simulink model "SimscapeCrane_MPChard"  (R2015b)
settings: Solver=ode15s  StartTime=0.0  StopTime=T  RelTol=1e-3
values from neighbouring files (symbols this model uses):
  m = m1/N    [ConstraintMatrices.m]
  N = N1/(n+c)    [SoftPadding.m]    (also in testMPC.m = ceil(Tf/Ts); testMyLP.m = ceil(1.5/Ts); testRHC.m = ceil(1.5/Ts))
  s = size(A)    [Prediction.m]
  Ts = 1.5/10    (= 0.15)    [testMPC.m]    (also in testMyLP.m; testRHC.m)
  xTarget = [xRange(2)*0.8 0 xRange(2)*0.8 0 0 0 0 0]'    [testMyLP.m]
  xZero = xRange(2)*0.05    [testMPC.m]    (also in testRHC.m = 0)
  yZero = yRange(2)*0.05    [testMPC.m]    (also in testRHC.m = 0)
undefined symbols (not defined in the file or in its folder): Al, blx0, blxe, CD, Dx0, MR, TxBreak, TxCoulomb, TxVisc, TyBreak, TyCoulomb, TzBreak, TzCoulomb, ucon, X, xRange, Y, yRange, Z, zRange, zZero
undefined symbols (not defined in the file): M, TorqueMultX, TorqueMultY, TorqueMultZ, TxTrans, TyTrans, TyVisc, TzTrans, TzVisc
libraries: sm_lib x146, fl_lib x62, nesl_utility x24, elec_lib x9, simulink x6, sm_double_wishbone_suspension_lib x4, aerolibtransform2 x1
(part 13 of 14)

== system SimscapeCrane_MPChard/Crane1/XY actuator/DC Y ==
  DCYcontrolSignal : Inport
  " Lead Screw" : fl_lib/Mechanical/Mechanisms/Wheel and Axle  R=2 cm  or=1  orient=1  t_specify=off  t_priority=High  t=0 N*m  f_specify=off  f_priority=High  f=0 N
  DC Motor2 : elec_lib/Actuators & Drivers/Rotational Actuators/DC Motor  parameterization=2  Ra=3.9 Ohm  La=1.2e-5 H  emf_or_torque=1  Kv=7.2e-5 V/rpm  Ki=6.876e-4 N*m/A  T_stall=10000 mN*m  w_max=190 rpm  w_rated=190 rpm  P_rated=0.08 W  V_rated=24 V  J=0.01 g*cm^2  lam_param=1  lam=0 N*m/(rad/s)  i_noload=0 A  V_i_noload=1.5 V  speed0=0 rpm  alpha=0.00393 1/K  Tmeas=25 C  thermal_mass=100 J/K  initial_temperature=25 C
  Force Sensor : fl_lib/Mechanical/Mechanical Sensors/Ideal Force Sensor
  Gear Box : fl_lib/Mechanical/Mechanisms/Gear Box  Tag=Factory Generic  ratio=1/30  t_in_specify=off  t_in_priority=High  t_in=0 N*m  t_out_specify=off  t_out_priority=High  t_out=0 N*m
  Mechanical Rotational Reference1 : fl_lib/Mechanical/Rotational Elements/Mechanical Rotational Reference
  Mechanical Translational Reference4 : fl_lib/Mechanical/Translational Elements/Mechanical Translational Reference
  PS Gain : fl_lib/Physical Signals/Functions/PS Gain  gain=-1*Uy
  PWM & H-Bridge1 : Subsystem
  SL2V_1 : Subsystem
  Conn1 : PMIOPort  Port=1  Side=Right
  wires:
  DCYcontrolSignal/1 -> SL2V_1/1(SL)
  connections:
  Force Sensor/RConn2 -- PS Gain/LConn1
  Mechanical Translational Reference4/LConn1 -- Force Sensor/LConn1
  Mechanical Rotational Reference1/LConn1 -- DC Motor2/RConn2
  Gear Box/RConn1 -- " Lead Screw"/LConn1
  Force Sensor/RConn1 -- " Lead Screw"/RConn1
  DC Motor2/LConn2 -- Gear Box/LConn1
  PWM & H-Bridge1/RConn2 -- DC Motor2/RConn1
  SL2V_1/RConn2 -- PWM & H-Bridge1/LConn2
  SL2V_1/RConn3 -- PWM & H-Bridge1/LConn3
  SL2V_1/RConn4 -- PWM & H-Bridge1/LConn4
  SL2V_1/RConn1 -- PWM & H-Bridge1/LConn1
  PWM & H-Bridge1/RConn1 -- DC Motor2/LConn1
  Conn1/RConn1 -- PS Gain/RConn1

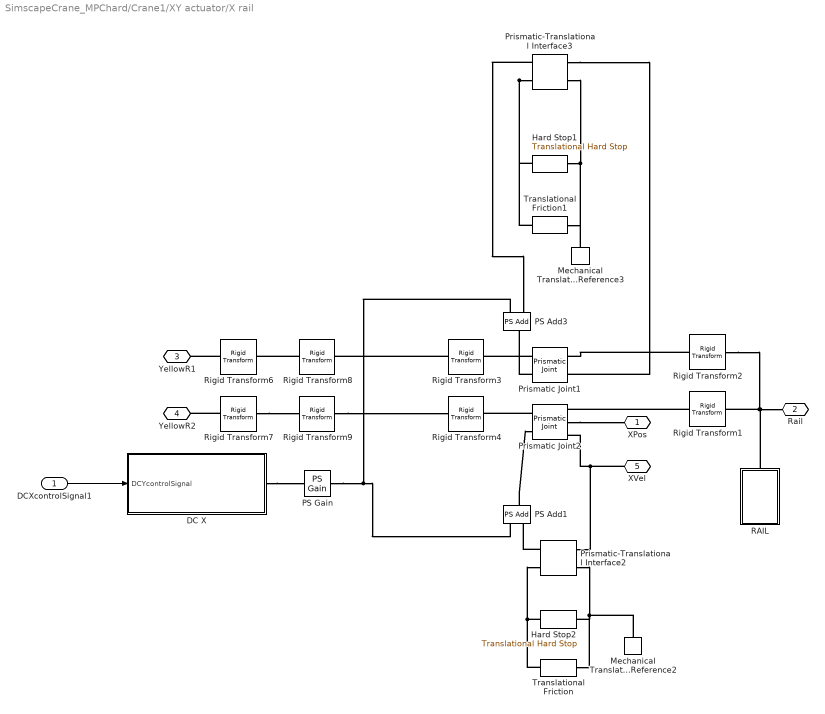
== system SimscapeCrane_MPChard/Crane1/XY actuator/X rail ==
  DCXcontrolSignal1 : Inport
  DC X : Subsystem
  Hard Stop1 : fl_lib/Mechanical/Translational Elements/Translational Hard Stop  upper_bnd=-xZero +xRange(2) m  lower_bnd=(xRange(1)-xZero) m  stiff_up=2e6 N/m  stiff_low=2e6 N/m  D_up=1000 N/(m/s)  D_low=1000 N/(m/s)  v_specify=off  v_priority=High  v=0 m/s  f_specify=off  f_priority=High  f=0 N  x_specify=off  x_priority=High  x=1 cm
  Hard Stop2 : fl_lib/Mechanical/Translational Elements/Translational Hard Stop  upper_bnd=-xZero +xRange(2) m  lower_bnd=(xRange(1)-xZero) m  stiff_up=2e6 N/m  stiff_low=2e6 N/m  D_up=1000 N/(m/s)  D_low=1000 N/(m/s)  v_specify=off  v_priority=High  v=0 m/s  f_specify=off  f_priority=High  f=0 N  x_specify=off  x_priority=High  x=1 cm
  Mechanical Translational Reference2 : fl_lib/Mechanical/Translational Elements/Mechanical Translational Reference
  Mechanical Translational Reference3 : fl_lib/Mechanical/Translational Elements/Mechanical Translational Reference
  PS Add1 : fl_lib/Physical Signals/Functions/PS Add
  PS Add3 : fl_lib/Physical Signals/Functions/PS Add
  PS Gain : fl_lib/Physical Signals/Functions/PS Gain  gain=1/2
  Prismatic Joint1 : sm_lib/Joints/Prismatic Joint  SenseConstraintForce=off  SenseConstraintForceX=off  SenseConstraintForceY=off  SenseConstraintForceZ=off  SenseConstraintTorque=off  SenseConstraintTorqueX=off  SenseConstraintTorqueY=off  SenseConstraintTorqueZ=off  SenseTotalForce=off  SenseTotalForceX=off  SenseTotalForceY=off  SenseTotalForceZ=off  SenseTotalTorque=off  SenseTotalTorqueX=off  SenseTotalTorqueY=off  SenseTotalTorqueZ=off  CompositeWrenchDir=FollowerOnBase  CompositeWrenchFrame=BaseFrame  EquilibriumPosition=0  EquilibriumPositionUnits=m  SpringStiffness=0  SpringStiffnessUnits=N/m  DampingCoefficient=0  DampingCoefficientUnits=N/(m/s)  TorqueActuationMode=InputTorque  MotionActuationMode=ComputedMotion  SensePosition=off  SenseVelocity=on  SenseAcceleration=off  SenseTorqueForce=off  PositionTargetSpecify=off  PositionTargetPriority=High  PositionTargetValue=0  PositionTargetValueUnits=m  VelocityTargetSpecify=off  VelocityTargetPriority=High  VelocityTargetValue=0  VelocityTargetValueUnits=m/s  BlockFunction=simmechanics.library.joints.prismatic_joint
  Prismatic Joint2 : sm_lib/Joints/Prismatic Joint  SenseConstraintForce=off  SenseConstraintForceX=off  SenseConstraintForceY=off  SenseConstraintForceZ=off  SenseConstraintTorque=off  SenseConstraintTorqueX=off  SenseConstraintTorqueY=off  SenseConstraintTorqueZ=off  SenseTotalForce=off  SenseTotalForceX=off  SenseTotalForceY=off  SenseTotalForceZ=off  SenseTotalTorque=off  SenseTotalTorqueX=off  SenseTotalTorqueY=off  SenseTotalTorqueZ=off  CompositeWrenchDir=FollowerOnBase  CompositeWrenchFrame=BaseFrame  EquilibriumPosition=0  EquilibriumPositionUnits=m  SpringStiffness=0  SpringStiffnessUnits=N/m  DampingCoefficient=0  DampingCoefficientUnits=N/(m/s)  TorqueActuationMode=InputTorque  MotionActuationMode=ComputedMotion  SensePosition=on  SenseVelocity=on  SenseAcceleration=off  SenseTorqueForce=off  PositionTargetSpecify=off  PositionTargetPriority=High  PositionTargetValue=0  PositionTargetValueUnits=m  VelocityTargetSpecify=off  VelocityTargetPriority=High  VelocityTargetValue=0  VelocityTargetValueUnits=m/s  BlockFunction=simmechanics.library.joints.prismatic_joint
  Prismatic-Translational Interface2 : sm_double_wishbone_suspension_lib/Testing Platform/Prismatic-Translational Interface
  Prismatic-Translational Interface3 : sm_double_wishbone_suspension_lib/Testing Platform/Prismatic-Translational Interface
  "RAIL " : Subsystem
  Rigid Transform1 : sm_lib/Frames and Transforms/Rigid Transform  TranslationMethod=Cartesian  TranslationLengthUnit=m  TranslationStandardAxis=+Z  TranslationStandardOffset=0  TranslationCartesianOffset="[0 0.5  0]"  TranslationROffset=0  TranslationROffsetUnits=m  TranslationZOffset=0  TranslationZOffsetUnits=m  TranslationThetaOffset=0  TranslationThetaOffsetUnits=deg  RotationMethod=StandardAxis  RotationAngleUnits=deg  RotationStandardAxis=-Y  RotationAngle=90  RotationArbitraryAxis=[0 0 1]  FollAlignAxisA=+X  BaseAlignAxisA=+Y  FollAlignAxisB=+Y  BaseAlignAxisB=+Z  RotationSequenceAxes=FollowerAxes  RotationSequence=XYX  RotationSequenceAngles=[0 0 0]  RotationSequenceAnglesUnits=deg  RotationMatrix=[1 0 0; 0 1 0; 0 0 1]  BlockFunction=simmechanics.library.frames_transforms.rigid_transform
  Rigid Transform2 : sm_lib/Frames and Transforms/Rigid Transform  TranslationMethod=Cartesian  TranslationLengthUnit=m  TranslationStandardAxis=+Z  TranslationStandardOffset=0  TranslationCartesianOffset="[ 0 -0.5  0]"  TranslationROffset=0  TranslationROffsetUnits=m  TranslationZOffset=0  TranslationZOffsetUnits=m  TranslationThetaOffset=0  TranslationThetaOffsetUnits=deg  RotationMethod=StandardAxis  RotationAngleUnits=deg  RotationStandardAxis=-Y  RotationAngle=90  RotationArbitraryAxis=[0 0 1]  FollAlignAxisA=+X  BaseAlignAxisA=+Y  FollAlignAxisB=+Y  BaseAlignAxisB=+Z  RotationSequenceAxes=FollowerAxes  RotationSequence=XYX  RotationSequenceAngles=[0 0 0]  RotationSequenceAnglesUnits=deg  RotationMatrix=[1 0 0; 0 1 0; 0 0 1]  BlockFunction=simmechanics.library.frames_transforms.rigid_transform
  Rigid Transform3 : sm_lib/Frames and Transforms/Rigid Transform  TranslationMethod=None  TranslationLengthUnit=m  TranslationStandardAxis=+Z  TranslationStandardOffset=0  TranslationCartesianOffset="[0.5 1  0]"  TranslationROffset=0  TranslationROffsetUnits=m  TranslationZOffset=0  TranslationZOffsetUnits=m  TranslationThetaOffset=0  TranslationThetaOffsetUnits=deg  RotationMethod=StandardAxis  RotationAngleUnits=deg  RotationStandardAxis=+Y  RotationAngle=90  RotationArbitraryAxis=[0 0 1]  FollAlignAxisA=+X  BaseAlignAxisA=+Y  FollAlignAxisB=+Y  BaseAlignAxisB=+Z  RotationSequenceAxes=FollowerAxes  RotationSequence=XYX  RotationSequenceAngles=[0 0 0]  RotationSequenceAnglesUnits=deg  RotationMatrix=[1 0 0; 0 1 0; 0 0 1]  BlockFunction=simmechanics.library.frames_transforms.rigid_transform
  Rigid Transform4 : sm_lib/Frames and Transforms/Rigid Transform  TranslationMethod=None  TranslationLengthUnit=m  TranslationStandardAxis=+Z  TranslationStandardOffset=0  TranslationCartesianOffset="[0.5 1  0]"  TranslationROffset=0  TranslationROffsetUnits=m  TranslationZOffset=0  TranslationZOffsetUnits=m  TranslationThetaOffset=0  TranslationThetaOffsetUnits=deg  RotationMethod=StandardAxis  RotationAngleUnits=deg  RotationStandardAxis=+Y  RotationAngle=90  RotationArbitraryAxis=[0 0 1]  FollAlignAxisA=+X  BaseAlignAxisA=+Y  FollAlignAxisB=+Y  BaseAlignAxisB=+Z  RotationSequenceAxes=FollowerAxes  RotationSequence=XYX  RotationSequenceAngles=[0 0 0]  RotationSequenceAnglesUnits=deg  RotationMatrix=[1 0 0; 0 1 0; 0 0 1]  BlockFunction=simmechanics.library.frames_transforms.rigid_transform
  Rigid Transform6 : sm_lib/Frames and Transforms/Rigid Transform  TranslationMethod=Cartesian  TranslationLengthUnit=m  TranslationStandardAxis=+Z  TranslationStandardOffset=0  TranslationCartesianOffset="[-0.28 0  0]"  TranslationROffset=0  TranslationROffsetUnits=m  TranslationZOffset=0  TranslationZOffsetUnits=m  TranslationThetaOffset=0  TranslationThetaOffsetUnits=deg  RotationMethod=None  RotationAngleUnits=deg  RotationStandardAxis=+Y  RotationAngle=90  RotationArbitraryAxis=[0 0 1]  FollAlignAxisA=+X  BaseAlignAxisA=+Y  FollAlignAxisB=+Y  BaseAlignAxisB=+Z  RotationSequenceAxes=FollowerAxes  RotationSequence=XYX  RotationSequenceAngles=[0 0 0]  RotationSequenceAnglesUnits=deg  RotationMatrix=[1 0 0; 0 1 0; 0 0 1]  BlockFunction=simmechanics.library.frames_transforms.rigid_transform
  Rigid Transform7 : sm_lib/Frames and Transforms/Rigid Transform  TranslationMethod=Cartesian  TranslationLengthUnit=m  TranslationStandardAxis=+Z  TranslationStandardOffset=0  TranslationCartesianOffset="[-0.28 0  0]"  TranslationROffset=0  TranslationROffsetUnits=m  TranslationZOffset=0  TranslationZOffsetUnits=m  TranslationThetaOffset=0  TranslationThetaOffsetUnits=deg  RotationMethod=None  RotationAngleUnits=deg  RotationStandardAxis=+Y  RotationAngle=90  RotationArbitraryAxis=[0 0 1]  FollAlignAxisA=+X  BaseAlignAxisA=+Y  FollAlignAxisB=+Y  BaseAlignAxisB=+Z  RotationSequenceAxes=FollowerAxes  RotationSequence=XYX  RotationSequenceAngles=[0 0 0]  RotationSequenceAnglesUnits=deg  RotationMatrix=[1 0 0; 0 1 0; 0 0 1]  BlockFunction=simmechanics.library.frames_transforms.rigid_transform
  Rigid Transform8 : sm_lib/Frames and Transforms/Rigid Transform  TranslationMethod=Cartesian  TranslationLengthUnit=m  TranslationStandardAxis=+Z  TranslationStandardOffset=0  TranslationCartesianOffset="[xZero 0  0]"  TranslationROffset=0  TranslationROffsetUnits=m  TranslationZOffset=0  TranslationZOffsetUnits=m  TranslationThetaOffset=0  TranslationThetaOffsetUnits=deg  RotationMethod=None  RotationAngleUnits=deg  RotationStandardAxis=+Y  RotationAngle=90  RotationArbitraryAxis=[0 0 1]  FollAlignAxisA=+X  BaseAlignAxisA=+Y  FollAlignAxisB=+Y  BaseAlignAxisB=+Z  RotationSequenceAxes=FollowerAxes  RotationSequence=XYX  RotationSequenceAngles=[0 0 0]  RotationSequenceAnglesUnits=deg  RotationMatrix=[1 0 0; 0 1 0; 0 0 1]  BlockFunction=simmechanics.library.frames_transforms.rigid_transform
  Rigid Transform9 : sm_lib/Frames and Transforms/Rigid Transform  TranslationMethod=Cartesian  TranslationLengthUnit=m  TranslationStandardAxis=+Z  TranslationStandardOffset=0  TranslationCartesianOffset="[xZero 0  0]"  TranslationROffset=0  TranslationROffsetUnits=m  TranslationZOffset=0  TranslationZOffsetUnits=m  TranslationThetaOffset=0  TranslationThetaOffsetUnits=deg  RotationMethod=None  RotationAngleUnits=deg  RotationStandardAxis=+Y  RotationAngle=90  RotationArbitraryAxis=[0 0 1]  FollAlignAxisA=+X  BaseAlignAxisA=+Y  FollAlignAxisB=+Y  BaseAlignAxisB=+Z  RotationSequenceAxes=FollowerAxes  RotationSequence=XYX  RotationSequenceAngles=[0 0 0]  RotationSequenceAnglesUnits=deg  RotationMatrix=[1 0 0; 0 1 0; 0 0 1]  BlockFunction=simmechanics.library.frames_transforms.rigid_transform
  Translational Friction : fl_lib/Mechanical/Translational Elements/Translational Friction  brkwy_frc=(TxBreak+TxCoulomb)/2 N  Col_frc=TxCoulomb/2 N  visc_coef=TxVisc/2 N/(m/s)  trans_coef=TxTrans s/m  vel_thr=1e-4 m/s  v_specify=off  v_priority=None  v=0 m/s  f_specify=off  f_priority=None  f=0 N
  Translational Friction1 : fl_lib/Mechanical/Translational Elements/Translational Friction  brkwy_frc=(TxBreak+TxCoulomb)/2 N  Col_frc=TxCoulomb/2 N  visc_coef=TxVisc/2 N/(m/s)  trans_coef=TxTrans s/m  vel_thr=1e-4 m/s  v_specify=off  v_priority=None  v=0 m/s  f_specify=off  f_priority=None  f=0 N
  XPos : PMIOPort  Port=1  Side=Right
  Rail : PMIOPort  Port=2  Side=Right
  YellowR1 : PMIOPort  Port=3  Side=Left
  YellowR2 : PMIOPort  Port=4  Side=Left
  XVel : PMIOPort  Port=5  Side=Right
  wires:
  DCXcontrolSignal1/1 -> DC X/1(DCYcontrolSignal)
  connections:
  Rigid Transform7/RConn1 -- Rigid Transform9/LConn1
  Rigid Transform6/LConn1 -- YellowR1/RConn1
  Prismatic Joint2/RConn2 -- XPos/RConn1
  Rigid Transform2/LConn1 -- Prismatic Joint1/RConn1
  Rigid Transform1/LConn1 -- Prismatic Joint2/RConn1
  "RAIL "/RConn1 -- Rigid Transform1/RConn1 -- Rigid Transform2/RConn1 -- Rail/RConn1
  Prismatic-Translational Interface2/LConn1 -- Prismatic Joint2/RConn3 -- XVel/RConn1
  Prismatic Joint1/LConn1 -- Rigid Transform3/RConn1
  Prismatic Joint2/LConn1 -- Rigid Transform4/RConn1
  PS Gain/RConn1 -- PS Add3/LConn2 -- PS Add1/LConn1
  DC X/RConn1 -- PS Gain/LConn1
  PS Add1/RConn1 -- Prismatic Joint2/LConn2
  Prismatic-Translational Interface2/RConn1 -- PS Add1/LConn2
  Prismatic Joint1/LConn2 -- PS Add3/RConn1
  Prismatic-Translational Interface3/LConn2 -- Hard Stop1/LConn1 -- Translational Friction1/LConn1 -- Mechanical Translational Reference3/LConn1
  Prismatic-Translational Interface3/RConn2 -- Hard Stop1/RConn1 -- Translational Friction1/RConn1
  Prismatic-Translational Interface3/RConn1 -- PS Add3/LConn1
  Prismatic-Translational Interface3/LConn1 -- Prismatic Joint1/RConn2
  Mechanical Translational Reference2/LConn1 -- Prismatic-Translational Interface2/LConn2 -- Hard Stop2/LConn1 -- Translational Friction/LConn1
  Hard Stop2/RConn1 -- Translational Friction/RConn1 -- Prismatic-Translational Interface2/RConn2
  Rigid Transform3/LConn1 -- Rigid Transform8/RConn1
  Rigid Transform7/LConn1 -- YellowR2/RConn1
  Rigid Transform8/LConn1 -- Rigid Transform6/RConn1
  Rigid Transform9/RConn1 -- Rigid Transform4/LConn1

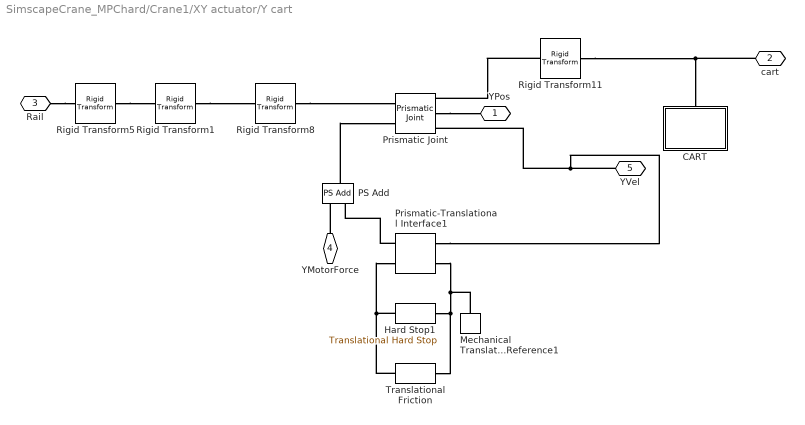
== system SimscapeCrane_MPChard/Crane1/XY actuator/Y cart ==
  CART : Subsystem
  Hard Stop1 : fl_lib/Mechanical/Translational Elements/Translational Hard Stop  upper_bnd=-yZero +yRange(2) m  lower_bnd=(yRange(1)-yZero) m  stiff_up=2e6 N/m  stiff_low=2e6 N/m  D_up=1000 N/(m/s)  D_low=1000 N/(m/s)  v_specify=off  v_priority=High  v=0 m/s  f_specify=off  f_priority=High  f=0 N  x_specify=off  x_priority=High  x=1 cm
  Mechanical Translational Reference1 : fl_lib/Mechanical/Translational Elements/Mechanical Translational Reference
  PS Add : fl_lib/Physical Signals/Functions/PS Add
  Prismatic Joint : sm_lib/Joints/Prismatic Joint  SenseConstraintForce=off  SenseConstraintForceX=off  SenseConstraintForceY=off  SenseConstraintForceZ=off  SenseConstraintTorque=off  SenseConstraintTorqueX=off  SenseConstraintTorqueY=off  SenseConstraintTorqueZ=off  SenseTotalForce=off  SenseTotalForceX=off  SenseTotalForceY=off  SenseTotalForceZ=off  SenseTotalTorque=off  SenseTotalTorqueX=off  SenseTotalTorqueY=off  SenseTotalTorqueZ=off  CompositeWrenchDir=BaseOnFollower  CompositeWrenchFrame=BaseFrame  EquilibriumPosition=0  EquilibriumPositionUnits=m  SpringStiffness=0  SpringStiffnessUnits=N/m  DampingCoefficient=0  DampingCoefficientUnits=N/(m/s)  TorqueActuationMode=InputTorque  MotionActuationMode=ComputedMotion  SensePosition=on  SenseVelocity=on  SenseAcceleration=off  SenseTorqueForce=off  PositionTargetSpecify=on  PositionTargetPriority=High  PositionTargetValue=0  PositionTargetValueUnits=m  VelocityTargetSpecify=off  VelocityTargetPriority=High  VelocityTargetValue=0  VelocityTargetValueUnits=m/s  BlockFunction=simmechanics.library.joints.prismatic_joint
  Prismatic-Translational Interface1 : sm_double_wishbone_suspension_lib/Testing Platform/Prismatic-Translational Interface
  Rigid Transform1 : sm_lib/Frames and Transforms/Rigid Transform  TranslationMethod=Cartesian  TranslationLengthUnit=m  TranslationStandardAxis=+Z  TranslationStandardOffset=0  TranslationCartesianOffset="[0 yZero  0]"  TranslationROffset=0  TranslationROffsetUnits=m  TranslationZOffset=0  TranslationZOffsetUnits=m  TranslationThetaOffset=0  TranslationThetaOffsetUnits=deg  RotationMethod=None  RotationAngleUnits=deg  RotationStandardAxis=+Y  RotationAngle=90  RotationArbitraryAxis=[0 0 1]  FollAlignAxisA=+X  BaseAlignAxisA=+Y  FollAlignAxisB=+Y  BaseAlignAxisB=+Z  RotationSequenceAxes=FollowerAxes  RotationSequence=XYX  RotationSequenceAngles=[0 0 0]  RotationSequenceAnglesUnits=deg  RotationMatrix=[1 0 0; 0 1 0; 0 0 1]  BlockFunction=simmechanics.library.frames_transforms.rigid_transform
  Rigid Transform11 : sm_lib/Frames and Transforms/Rigid Transform  TranslationMethod=None  TranslationLengthUnit=m  TranslationStandardAxis=+Z  TranslationStandardOffset=0  TranslationCartesianOffset="[-0.5 0  0]"  TranslationROffset=0  TranslationROffsetUnits=m  TranslationZOffset=0  TranslationZOffsetUnits=m  TranslationThetaOffset=0  TranslationThetaOffsetUnits=deg  RotationMethod=StandardAxis  RotationAngleUnits=deg  RotationStandardAxis=+X  RotationAngle=90  RotationArbitraryAxis=[0 0 1]  FollAlignAxisA=+X  BaseAlignAxisA=+Y  FollAlignAxisB=+Y  BaseAlignAxisB=+Z  RotationSequenceAxes=FollowerAxes  RotationSequence=XYX  RotationSequenceAngles=[0 0 0]  RotationSequenceAnglesUnits=deg  RotationMatrix=[1 0 0; 0 1 0; 0 0 1]  BlockFunction=simmechanics.library.frames_transforms.rigid_transform
  Rigid Transform5 : sm_lib/Frames and Transforms/Rigid Transform  TranslationMethod=Cartesian  TranslationLengthUnit=m  TranslationStandardAxis=+Z  TranslationStandardOffset=0  TranslationCartesianOffset="[0 -0.3  0]"  TranslationROffset=0  TranslationROffsetUnits=m  TranslationZOffset=0  TranslationZOffsetUnits=m  TranslationThetaOffset=0  TranslationThetaOffsetUnits=deg  RotationMethod=None  RotationAngleUnits=deg  RotationStandardAxis=+Y  RotationAngle=90  RotationArbitraryAxis=[0 0 1]  FollAlignAxisA=+X  BaseAlignAxisA=+Y  FollAlignAxisB=+Y  BaseAlignAxisB=+Z  RotationSequenceAxes=FollowerAxes  RotationSequence=XYX  RotationSequenceAngles=[0 0 0]  RotationSequenceAnglesUnits=deg  RotationMatrix=[1 0 0; 0 1 0; 0 0 1]  BlockFunction=simmechanics.library.frames_transforms.rigid_transform
  Rigid Transform8 : sm_lib/Frames and Transforms/Rigid Transform  TranslationMethod=None  TranslationLengthUnit=m  TranslationStandardAxis=+Z  TranslationStandardOffset=0  TranslationCartesianOffset="[-0.5 0  0]"  TranslationROffset=0  TranslationROffsetUnits=m  TranslationZOffset=0  TranslationZOffsetUnits=m  TranslationThetaOffset=0  TranslationThetaOffsetUnits=deg  RotationMethod=StandardAxis  RotationAngleUnits=deg  RotationStandardAxis=-X  RotationAngle=90  RotationArbitraryAxis=[0 0 1]  FollAlignAxisA=+X  BaseAlignAxisA=+Y  FollAlignAxisB=+Y  BaseAlignAxisB=+Z  RotationSequenceAxes=FollowerAxes  RotationSequence=XYX  RotationSequenceAngles=[0 0 0]  RotationSequenceAnglesUnits=deg  RotationMatrix=[1 0 0; 0 1 0; 0 0 1]  BlockFunction=simmechanics.library.frames_transforms.rigid_transform
  Translational Friction : fl_lib/Mechanical/Translational Elements/Translational Friction  brkwy_frc=TyBreak+TyCoulomb N  Col_frc=TyCoulomb N  visc_coef=TyVisc N/(m/s)  trans_coef=TyTrans s/m  vel_thr=1e-4 m/s  v_specify=off  v_priority=None  v=0 m/s  f_specify=off  f_priority=None  f=0 N
  YPos : PMIOPort  Port=1  Side=Right
  cart : PMIOPort  Port=2  Side=Right
  Rail : PMIOPort  Port=3  Side=Left
  YMotorForce : PMIOPort  Port=4  Side=Left
  YVel : PMIOPort  Port=5  Side=Right
  connections:
  Rail/RConn1 -- Rigid Transform5/LConn1
  Prismatic Joint/RConn2 -- YPos/RConn1
  Rigid Transform11/RConn1 -- cart/RConn1 -- CART/RConn1
  Rigid Transform8/RConn1 -- Prismatic Joint/LConn1
  Rigid Transform11/LConn1 -- Prismatic Joint/RConn1
  YVel/RConn1 -- Prismatic-Translational Interface1/LConn1 -- Prismatic Joint/RConn3
  YMotorForce/RConn1 -- PS Add/LConn1
  PS Add/RConn1 -- Prismatic Joint/LConn2
  Translational Friction/RConn1 -- Hard Stop1/RConn1 -- Prismatic-Translational Interface1/RConn2
  Prismatic-Translational Interface1/LConn2 -- Hard Stop1/LConn1 -- Translational Friction/LConn1 -- Mechanical Translational Reference1/LConn1
  Prismatic-Translational Interface1/RConn1 -- PS Add/LConn2
  Rigid Transform1/RConn1 -- Rigid Transform8/LConn1
  Rigid Transform5/RConn1 -- Rigid Transform1/LConn1

== system SimscapeCrane_MPChard/Crane1/Frame/XMotorAesthetics/Motor ==
  Cart2 : sm_lib/Body Elements/Solid  InertiaType=PointMass  Mass=0  MassUnits=kg  CenterOfMass=[0 0 0]  CenterOfMassUnits=m  MomentsOfInertia=[1 1 1]  MomentsOfInertiaUnits=kg*m^2  ProductsOfInertia=[0 0 0]  ProductsOfInertiaUnits=kg*m^2  DensityBased=off  Density=1000  DensityUnits=kg/(m^3)  DoExposeReferenceFrame=on  SerializedFrames=<Frames/>  GraphicType=FromGeometry  MarkerShape=Sphere  MarkerSize=10  MarkerSizeUnits=m  GraphicVisPropType=AdvancedVisualProperties  GraphicDiffuseColor=[0.1 0.1 0.0]  GraphicSpecularColor=[0.5 0.5 0.5 1.0]  GraphicAmbientColor=[0.15 0.2 0.3 1.0]  GraphicEmissiveColor=[0.0 0.0 0.0 1.0]  GraphicShininess=30  GraphicOpacity=1.0  GeometryShape=Cylinder  RectangleSize=[1 1]  RectangleSizeUnits=m  BrickDimensions=[0.06 0.12 0.12]  BrickDimensionUnits=m  CylinderRadius=1.7  CylinderRadiusUnits=cm  CylinderLength=6  CylinderLengthUnits=cm  SphereRadius=1  SphereRadiusUnits=m  EllipsoidRadii=[1 1 1]  EllipsoidRadiiUnits=m  ExtrusionCrossSection=[1 1; -1 1; -1 -1; 1 -1]  ExtrusionCrossSectionUnits=m  ExtrusionLength=1  ExtrusionLengthUnits=m  PolygonNumSides=3  PolygonOuterRadius=1  PolygonOuterRadiusUnits=m  ExtGeomFileType=STL  ExtGeomFileUnits=m  RevolutionCrossSection=[1 1; 1 -1; 2 -1; 2 1]  RevolutionCrossSectionUnits=m  RevolutionExtent=Full  RevolutionAngle=180  RevolutionAngleUnits=deg  BlockFunction=simmechanics.library.body_elements.solid
  Cart3 : sm_lib/Body Elements/Solid  InertiaType=PointMass  Mass=0  MassUnits=kg  CenterOfMass=[0 0 0]  CenterOfMassUnits=m  MomentsOfInertia=[1 1 1]  MomentsOfInertiaUnits=kg*m^2  ProductsOfInertia=[0 0 0]  ProductsOfInertiaUnits=kg*m^2  DensityBased=off  Density=1000  DensityUnits=kg/(m^3)  DoExposeReferenceFrame=on  SerializedFrames=<Frames/>  GraphicType=FromGeometry  MarkerShape=Sphere  MarkerSize=10  MarkerSizeUnits=m  GraphicVisPropType=SimpleVisualProperties  GraphicDiffuseColor=[0.4 0.4 0.4]  GraphicSpecularColor=[0.5 0.5 0.5 1.0]  GraphicAmbientColor=[0.15 0.15 0.15 1.0]  GraphicEmissiveColor=[0.0 0.0 0.0 1.0]  GraphicShininess=75  GraphicOpacity=1.0  GeometryShape=Cylinder  RectangleSize=[1 1]  RectangleSizeUnits=m  BrickDimensions=[0.06 0.12 0.12]  BrickDimensionUnits=m  CylinderRadius=2.6  CylinderRadiusUnits=cm  CylinderLength=3  CylinderLengthUnits=cm  SphereRadius=1  SphereRadiusUnits=m  EllipsoidRadii=[1 1 1]  EllipsoidRadiiUnits=m  ExtrusionCrossSection=[1 1; -1 1; -1 -1; 1 -1]  ExtrusionCrossSectionUnits=m  ExtrusionLength=1  ExtrusionLengthUnits=m  PolygonNumSides=3  PolygonOuterRadius=1  PolygonOuterRadiusUnits=m  ExtGeomFileType=STL  ExtGeomFileUnits=m  RevolutionCrossSection=[1 1; 1 -1; 2 -1; 2 1]  RevolutionCrossSectionUnits=m  RevolutionExtent=Full  RevolutionAngle=180  RevolutionAngleUnits=deg  BlockFunction=simmechanics.library.body_elements.solid
  Rigid Transform3 : sm_lib/Frames and Transforms/Rigid Transform  TranslationMethod=None  TranslationLengthUnit=m  TranslationStandardAxis=-X  TranslationStandardOffset=0.04  TranslationCartesianOffset="[-0.5 0  0]"  TranslationROffset=0  TranslationROffsetUnits=m  TranslationZOffset=0  TranslationZOffsetUnits=m  TranslationThetaOffset=0  TranslationThetaOffsetUnits=deg  RotationMethod=StandardAxis  RotationAngleUnits=deg  RotationStandardAxis=-X  RotationAngle=90  RotationArbitraryAxis=[0 0 1]  FollAlignAxisA=+X  BaseAlignAxisA=+Y  FollAlignAxisB=+Y  BaseAlignAxisB=+Z  RotationSequenceAxes=FollowerAxes  RotationSequence=XYX  RotationSequenceAngles=[0 0 0]  RotationSequenceAnglesUnits=deg  RotationMatrix=[1 0 0; 0 1 0; 0 0 1]  BlockFunction=simmechanics.library.frames_transforms.rigid_transform
  Rigid Transform4 : sm_lib/Frames and Transforms/Rigid Transform  TranslationMethod=None  TranslationLengthUnit=m  TranslationStandardAxis=-X  TranslationStandardOffset=0.04  TranslationCartesianOffset="[-0.5 0  0]"  TranslationROffset=0  TranslationROffsetUnits=m  TranslationZOffset=0  TranslationZOffsetUnits=m  TranslationThetaOffset=0  TranslationThetaOffsetUnits=deg  RotationMethod=StandardAxis  RotationAngleUnits=deg  RotationStandardAxis=-X  RotationAngle=90  RotationArbitraryAxis=[0 0 1]  FollAlignAxisA=+X  BaseAlignAxisA=+Y  FollAlignAxisB=+Y  BaseAlignAxisB=+Z  RotationSequenceAxes=FollowerAxes  RotationSequence=XYX  RotationSequenceAngles=[0 0 0]  RotationSequenceAnglesUnits=deg  RotationMatrix=[1 0 0; 0 1 0; 0 0 1]  BlockFunction=simmechanics.library.frames_transforms.rigid_transform
  Rigid Transform5 : sm_lib/Frames and Transforms/Rigid Transform  TranslationMethod=StandardAxis  TranslationLengthUnit=m  TranslationStandardAxis=-Y  TranslationStandardOffset=0.015  TranslationCartesianOffset="[-0.5 0  0]"  TranslationROffset=0  TranslationROffsetUnits=m  TranslationZOffset=0  TranslationZOffsetUnits=m  TranslationThetaOffset=0  TranslationThetaOffsetUnits=deg  RotationMethod=None  RotationAngleUnits=deg  RotationStandardAxis=-X  RotationAngle=90  RotationArbitraryAxis=[0 0 1]  FollAlignAxisA=+X  BaseAlignAxisA=+Y  FollAlignAxisB=+Y  BaseAlignAxisB=+Z  RotationSequenceAxes=FollowerAxes  RotationSequence=XYX  RotationSequenceAngles=[0 0 0]  RotationSequenceAnglesUnits=deg  RotationMatrix=[1 0 0; 0 1 0; 0 0 1]  BlockFunction=simmechanics.library.frames_transforms.rigid_transform
  Rigid Transform6 : sm_lib/Frames and Transforms/Rigid Transform  TranslationMethod=StandardAxis  TranslationLengthUnit=m  TranslationStandardAxis=+Y  TranslationStandardOffset=0.03  TranslationCartesianOffset="[-0.5 0  0]"  TranslationROffset=0  TranslationROffsetUnits=m  TranslationZOffset=0  TranslationZOffsetUnits=m  TranslationThetaOffset=0  TranslationThetaOffsetUnits=deg  RotationMethod=None  RotationAngleUnits=deg  RotationStandardAxis=-X  RotationAngle=90  RotationArbitraryAxis=[0 0 1]  FollAlignAxisA=+X  BaseAlignAxisA=+Y  FollAlignAxisB=+Y  BaseAlignAxisB=+Z  RotationSequenceAxes=FollowerAxes  RotationSequence=XYX  RotationSequenceAngles=[0 0 0]  RotationSequenceAnglesUnits=deg  RotationMatrix=[1 0 0; 0 1 0; 0 0 1]  BlockFunction=simmechanics.library.frames_transforms.rigid_transform
  Conn1 : PMIOPort  Port=1  Side=Left
  connections:
  Rigid Transform3/RConn1 -- Cart2/RConn1
  Rigid Transform4/RConn1 -- Cart3/RConn1
  Rigid Transform5/LConn1 -- Rigid Transform6/LConn1 -- Conn1/RConn1
  Rigid Transform6/RConn1 -- Rigid Transform4/LConn1
  Rigid Transform5/RConn1 -- Rigid Transform3/LConn1

== system SimscapeCrane_MPChard/Crane1/XY actuator/DC Y/PWM & H-Bridge1 ==
  note: For validation purposes the simulation mode
      | can be set to PWM in both the Controlled PWM
      | and H-Bridge blocks.
  Controlled PWM Voltage : elec_lib/Actuators & Drivers/Drivers/Controlled PWM Voltage  F=10000 Hz  TD=0 s  pulse_width_offset=0 s  Vmin=0 V  Vmax=5 V  Vm=5 V  pwm_or_av=2  event_type=1  sample_time=1e-6 s
  Electrical Reference2 : fl_lib/Electrical/Electrical Elements/Electrical Reference
  H-Bridge : elec_lib/Actuators & Drivers/Drivers/H-Bridge  Venable=2.5 V  Vmax=5 V  Vreverse=2.5 V  Vbrake=2.5 V  Vm=24 V  pwm_or_av=2  discontinuous=0  freewheeling_mode=1  freewheeling_mode_disc=1  Ron=0.1 Ohm  Don=0.1 Ohm  Rload=10 Ohm  Lload=1e-5 H  F=10 kHz  thermal_mass=100 J/K  initial_temperature=298.15 K  Ron2=0.1 Ohm  Don2=0.05 Ohm  Tmeas=298.15 K  Tmeas2=398.15 K
  PWM Scope : Subsystem  Commented=on
  REV Scope : Subsystem  Commented=on
  Vr Scope : Subsystem  Commented=on
  V+ : PMIOPort  Port=1  Side=Right
  V- : PMIOPort  Port=2  Side=Right
  Vr : PMIOPort  Port=3  Side=Left
  REV : PMIOPort  Port=4  Side=Left
  "brk " : PMIOPort  Port=5  Side=Left
  "gnd " : PMIOPort  Port=6  Side=Left
  connections:
  V+/RConn1 -- H-Bridge/RConn1
  H-Bridge/RConn2 -- V-/RConn1 -- Electrical Reference2/LConn1
  PWM Scope/LConn1 -- H-Bridge/LConn1 -- Controlled PWM Voltage/RConn1
  Vr Scope/LConn1 -- Controlled PWM Voltage/LConn1 -- Vr/RConn1
  REV Scope/LConn1 -- H-Bridge/LConn3 -- REV/RConn1
  "gnd "/RConn1 -- H-Bridge/LConn2 -- Controlled PWM Voltage/RConn2 -- Controlled PWM Voltage/LConn2
  "brk "/RConn1 -- H-Bridge/LConn4

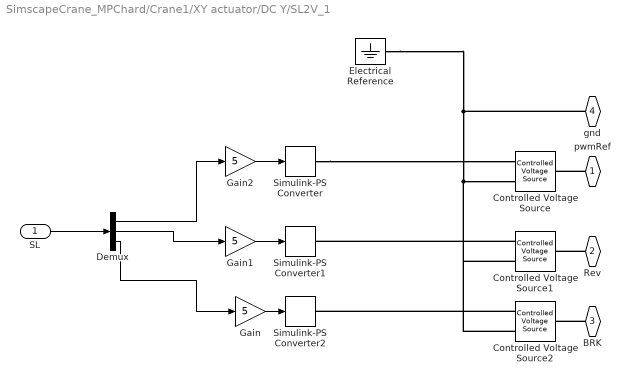
== system SimscapeCrane_MPChard/Crane1/XY actuator/DC Y/SL2V_1 ==
  SL : Inport
  Controlled Voltage Source : fl_lib/Electrical/Electrical Sources/Controlled Voltage Source
  Controlled Voltage Source1 : fl_lib/Electrical/Electrical Sources/Controlled Voltage Source
  Controlled Voltage Source2 : fl_lib/Electrical/Electrical Sources/Controlled Voltage Source
  Demux : Demux  Outputs=3
  Electrical Reference : fl_lib/Electrical/Electrical Elements/Electrical Reference
  Gain : Gain  Gain=5
  Gain1 : Gain  Gain=5
  Gain2 : Gain  Gain=5
  Simulink-PS Converter : nesl_utility/Simulink-PS Converter  PhysicalDomain=network_engine_domain  SubClassName=ps_input  LeftPortType=input  RightPortType=output  PseudoPeriodic=off  Frequencies=[]  NoiseDistribution=none  NoiseParameters=[]  Unit=V  AffineConversion=off  InputFiltering=off  SimscapeFilterOrder=1  InputFilterTimeConstant=.001  UdotUserProvided=0
  Simulink-PS Converter1 : nesl_utility/Simulink-PS Converter  PhysicalDomain=network_engine_domain  SubClassName=ps_input  LeftPortType=input  RightPortType=output  PseudoPeriodic=off  Frequencies=[]  NoiseDistribution=none  NoiseParameters=[]  Unit=V  AffineConversion=off  InputFiltering=off  SimscapeFilterOrder=1  InputFilterTimeConstant=.001  UdotUserProvided=0
  Simulink-PS Converter2 : nesl_utility/Simulink-PS Converter  PhysicalDomain=network_engine_domain  SubClassName=ps_input  LeftPortType=input  RightPortType=output  PseudoPeriodic=off  Frequencies=[]  NoiseDistribution=none  NoiseParameters=[]  Unit=V  AffineConversion=off  InputFiltering=off  SimscapeFilterOrder=1  InputFilterTimeConstant=.001  UdotUserProvided=0
  pwmRef : PMIOPort  Port=1  Side=Right
  Rev : PMIOPort  Port=2  Side=Right
  BRK : PMIOPort  Port=3  Side=Right
  "gnd " : PMIOPort  Port=4  Side=Right
  wires:
  SL/1 -> Demux/1
  Demux/1 -> Gain2/1
  Demux/3 -> Gain/1
  Gain/1 -> Simulink-PS Converter2/1
  Demux/2 -> Gain1/1
  Gain1/1 -> Simulink-PS Converter1/1
  Gain2/1 -> Simulink-PS Converter/1
  connections:
  Simulink-PS Converter/RConn1 -- Controlled Voltage Source/RConn1
  pwmRef/RConn1 -- Controlled Voltage Source/LConn1
  Electrical Reference/LConn1 -- Controlled Voltage Source/RConn2 -- Controlled Voltage Source1/RConn2 -- Controlled Voltage Source2/RConn2 -- "gnd "/RConn1
  Rev/RConn1 -- Controlled Voltage Source1/LConn1
  Controlled Voltage Source2/RConn1 -- Simulink-PS Converter2/RConn1
  BRK/RConn1 -- Controlled Voltage Source2/LConn1
  Controlled Voltage Source1/RConn1 -- Simulink-PS Converter1/RConn1

== system SimscapeCrane_MPChard/Crane1/XY actuator/X rail/DC X ==
  DCYcontrolSignal : Inport
  " Lead Screw" : fl_lib/Mechanical/Mechanisms/Wheel and Axle  R=2 cm  or=1  orient=1  t_specify=off  t_priority=High  t=0 N*m  f_specify=off  f_priority=High  f=0 N
  DC Motor2 : elec_lib/Actuators & Drivers/Rotational Actuators/DC Motor  parameterization=2  Ra=3.9 Ohm  La=1.2e-5 H  emf_or_torque=1  Kv=7.2e-5 V/rpm  Ki=6.876e-4 N*m/A  T_stall=10000 mN*m  w_max=190 rpm  w_rated=190 rpm  P_rated=0.08 W  V_rated=24 V  J=0.01 g*cm^2  lam_param=1  lam=0 N*m/(rad/s)  i_noload=0 A  V_i_noload=1.5 V  speed0=0 rpm  alpha=0.00393 1/K  Tmeas=25 C  thermal_mass=100 J/K  initial_temperature=25 C
  Force Sensor : fl_lib/Mechanical/Mechanical Sensors/Ideal Force Sensor
  Gear Box : fl_lib/Mechanical/Mechanisms/Gear Box  Tag=Factory Generic  ratio=1/30  t_in_specify=off  t_in_priority=High  t_in=0 N*m  t_out_specify=off  t_out_priority=High  t_out=0 N*m
  Mechanical Rotational Reference1 : fl_lib/Mechanical/Rotational Elements/Mechanical Rotational Reference
  Mechanical Translational Reference4 : fl_lib/Mechanical/Translational Elements/Mechanical Translational Reference
  PS Gain : fl_lib/Physical Signals/Functions/PS Gain  gain=-1*Ux
  PWM & H-Bridge : Subsystem
  SL2V_2 : Subsystem
  Conn1 : PMIOPort  Port=1  Side=Right
  wires:
  DCYcontrolSignal/1 -> SL2V_2/1(SL)
  connections:
  PS Gain/RConn1 -- Conn1/RConn1
  Mechanical Translational Reference4/LConn1 -- Force Sensor/LConn1
  Mechanical Rotational Reference1/LConn1 -- DC Motor2/RConn2
  Gear Box/RConn1 -- " Lead Screw"/LConn1
  Force Sensor/RConn1 -- " Lead Screw"/RConn1
  DC Motor2/LConn2 -- Gear Box/LConn1
  PWM & H-Bridge/RConn1 -- DC Motor2/LConn1
  PWM & H-Bridge/RConn2 -- DC Motor2/RConn1
  SL2V_2/RConn2 -- PWM & H-Bridge/LConn2
  SL2V_2/RConn3 -- PWM & H-Bridge/LConn3
  SL2V_2/RConn1 -- PWM & H-Bridge/LConn1
  SL2V_2/RConn4 -- PWM & H-Bridge/LConn4
  Force Sensor/RConn2 -- PS Gain/LConn1

== system SimscapeCrane_MPChard/Crane1/XY actuator/X rail/RAIL  ==
  Aesthetics : Subsystem
  Rail : sm_lib/Body Elements/Solid  InertiaType=CalculateFromGeometry  Mass=MR/2  MassUnits=kg  CenterOfMass=[0 0 0]  CenterOfMassUnits=m  MomentsOfInertia=[1 1 1]  MomentsOfInertiaUnits=kg*m^2  ProductsOfInertia=[0 0 0]  ProductsOfInertiaUnits=kg*m^2  DensityBased=off  Density=1000  DensityUnits=kg/(m^3)  DoExposeReferenceFrame=on  SerializedFrames=<Frames/>  GraphicType=FromGeometry  MarkerShape=Sphere  MarkerSize=10  MarkerSizeUnits=m  GraphicVisPropType=AdvancedVisualProperties  GraphicDiffuseColor=[0.0 0.0 0.0]  GraphicSpecularColor=[0.5 0.5 0.5 1.0]  GraphicAmbientColor=[0.15 0.15 0.15 1.0]  GraphicEmissiveColor=[0.0 0.0 0.0 1.0]  GraphicShininess=100  GraphicOpacity=1.0  GeometryShape=Brick  RectangleSize=[1 1]  RectangleSizeUnits=m  BrickDimensions=[1.2 0.04 0.04]  BrickDimensionUnits=m  CylinderRadius=0.02  CylinderRadiusUnits=m  CylinderLength=1  CylinderLengthUnits=m  SphereRadius=1  SphereRadiusUnits=m  EllipsoidRadii=[1 1 1]  EllipsoidRadiiUnits=m  ExtrusionCrossSection=[1 1; -1 1; -1 -1; 1 -1]  ExtrusionCrossSectionUnits=m  ExtrusionLength=1  ExtrusionLengthUnits=m  PolygonNumSides=3  PolygonOuterRadius=1  PolygonOuterRadiusUnits=m  ExtGeomFileType=STL  ExtGeomFileUnits=m  RevolutionCrossSection=[1 1; 1 -1; 2 -1; 2 1]  RevolutionCrossSectionUnits=m  RevolutionExtent=Full  RevolutionAngle=180  RevolutionAngleUnits=deg  BlockFunction=simmechanics.library.body_elements.solid
  Rail1 : sm_lib/Body Elements/Solid  InertiaType=CalculateFromGeometry  Mass=MR/2  MassUnits=kg  CenterOfMass=[0 0 0]  CenterOfMassUnits=m  MomentsOfInertia=[1 1 1]  MomentsOfInertiaUnits=kg*m^2  ProductsOfInertia=[0 0 0]  ProductsOfInertiaUnits=kg*m^2  DensityBased=off  Density=1000  DensityUnits=kg/(m^3)  DoExposeReferenceFrame=on  SerializedFrames=<Frames/>  GraphicType=FromGeometry  MarkerShape=Sphere  MarkerSize=10  MarkerSizeUnits=m  GraphicVisPropType=AdvancedVisualProperties  GraphicDiffuseColor=[0.0 0.0 0.0]  GraphicSpecularColor=[0.5 0.5 0.5 1.0]  GraphicAmbientColor=[0.15 0.15 0.15 1.0]  GraphicEmissiveColor=[0.0 0.0 0.0 1.0]  GraphicShininess=100  GraphicOpacity=1.0  GeometryShape=Brick  RectangleSize=[1 1]  RectangleSizeUnits=m  BrickDimensions=[1.2 0.04 0.04]  BrickDimensionUnits=m  CylinderRadius=0.02  CylinderRadiusUnits=m  CylinderLength=1  CylinderLengthUnits=m  SphereRadius=1  SphereRadiusUnits=m  EllipsoidRadii=[1 1 1]  EllipsoidRadiiUnits=m  ExtrusionCrossSection=[1 1; -1 1; -1 -1; 1 -1]  ExtrusionCrossSectionUnits=m  ExtrusionLength=1  ExtrusionLengthUnits=m  PolygonNumSides=3  PolygonOuterRadius=1  PolygonOuterRadiusUnits=m  ExtGeomFileType=STL  ExtGeomFileUnits=m  RevolutionCrossSection=[1 1; 1 -1; 2 -1; 2 1]  RevolutionCrossSectionUnits=m  RevolutionExtent=Full  RevolutionAngle=180  RevolutionAngleUnits=deg  BlockFunction=simmechanics.library.body_elements.solid
  Rigid Transform1 : sm_lib/Frames and Transforms/Rigid Transform  TranslationMethod=StandardAxis  TranslationLengthUnit=m  TranslationStandardAxis=-X  TranslationStandardOffset=0.04  TranslationCartesianOffset="[-0.5 0  0]"  TranslationROffset=0  TranslationROffsetUnits=m  TranslationZOffset=0  TranslationZOffsetUnits=m  TranslationThetaOffset=0  TranslationThetaOffsetUnits=deg  RotationMethod=None  RotationAngleUnits=deg  RotationStandardAxis=+Y  RotationAngle=90  RotationArbitraryAxis=[0 0 1]  FollAlignAxisA=+X  BaseAlignAxisA=+Y  FollAlignAxisB=+Y  BaseAlignAxisB=+Z  RotationSequenceAxes=FollowerAxes  RotationSequence=XYX  RotationSequenceAngles=[0 0 0]  RotationSequenceAnglesUnits=deg  RotationMatrix=[1 0 0; 0 1 0; 0 0 1]  BlockFunction=simmechanics.library.frames_transforms.rigid_transform
  Rigid Transform2 : sm_lib/Frames and Transforms/Rigid Transform  TranslationMethod=StandardAxis  TranslationLengthUnit=m  TranslationStandardAxis=+X  TranslationStandardOffset=0.04  TranslationCartesianOffset="[-0.5 0  0]"  TranslationROffset=0  TranslationROffsetUnits=m  TranslationZOffset=0  TranslationZOffsetUnits=m  TranslationThetaOffset=0  TranslationThetaOffsetUnits=deg  RotationMethod=None  RotationAngleUnits=deg  RotationStandardAxis=+Y  RotationAngle=90  RotationArbitraryAxis=[0 0 1]  FollAlignAxisA=+X  BaseAlignAxisA=+Y  FollAlignAxisB=+Y  BaseAlignAxisB=+Z  RotationSequenceAxes=FollowerAxes  RotationSequence=XYX  RotationSequenceAngles=[0 0 0]  RotationSequenceAnglesUnits=deg  RotationMatrix=[1 0 0; 0 1 0; 0 0 1]  BlockFunction=simmechanics.library.frames_transforms.rigid_transform
  Rigid Transform3 : sm_lib/Frames and Transforms/Rigid Transform  TranslationMethod=StandardAxis  TranslationLengthUnit=m  TranslationStandardAxis=-Z  TranslationStandardOffset=0.04  TranslationCartesianOffset="[-0.5 0  0]"  TranslationROffset=0  TranslationROffsetUnits=m  TranslationZOffset=0  TranslationZOffsetUnits=m  TranslationThetaOffset=0  TranslationThetaOffsetUnits=deg  RotationMethod=None  RotationAngleUnits=deg  RotationStandardAxis=+Y  RotationAngle=90  RotationArbitraryAxis=[0 0 1]  FollAlignAxisA=+X  BaseAlignAxisA=+Y  FollAlignAxisB=+Y  BaseAlignAxisB=+Z  RotationSequenceAxes=FollowerAxes  RotationSequence=XYX  RotationSequenceAngles=[0 0 0]  RotationSequenceAnglesUnits=deg  RotationMatrix=[1 0 0; 0 1 0; 0 0 1]  BlockFunction=simmechanics.library.frames_transforms.rigid_transform
  Rigid Transform5 : sm_lib/Frames and Transforms/Rigid Transform  TranslationMethod=None  TranslationLengthUnit=m  TranslationStandardAxis=-Z  TranslationStandardOffset=0.04  TranslationCartesianOffset="[-0.5 0  0]"  TranslationROffset=0  TranslationROffsetUnits=m  TranslationZOffset=0  TranslationZOffsetUnits=m  TranslationThetaOffset=0  TranslationThetaOffsetUnits=deg  RotationMethod=StandardAxis  RotationAngleUnits=deg  RotationStandardAxis=+Z  RotationAngle=90  RotationArbitraryAxis=[0 0 1]  FollAlignAxisA=+X  BaseAlignAxisA=+Y  FollAlignAxisB=+Y  BaseAlignAxisB=+Z  RotationSequenceAxes=FollowerAxes  RotationSequence=XYX  RotationSequenceAngles=[0 0 0]  RotationSequenceAnglesUnits=deg  RotationMatrix=[1 0 0; 0 1 0; 0 0 1]  BlockFunction=simmechanics.library.frames_transforms.rigid_transform
  Rigid Transform6 : sm_lib/Frames and Transforms/Rigid Transform  TranslationMethod=None  TranslationLengthUnit=m  TranslationStandardAxis=-Z  TranslationStandardOffset=0.04  TranslationCartesianOffset="[-0.5 0  0]"  TranslationROffset=0  TranslationROffsetUnits=m  TranslationZOffset=0  TranslationZOffsetUnits=m  TranslationThetaOffset=0  TranslationThetaOffsetUnits=deg  RotationMethod=StandardAxis  RotationAngleUnits=deg  RotationStandardAxis=+Z  RotationAngle=90  RotationArbitraryAxis=[0 0 1]  FollAlignAxisA=+X  BaseAlignAxisA=+Y  FollAlignAxisB=+Y  BaseAlignAxisB=+Z  RotationSequenceAxes=FollowerAxes  RotationSequence=XYX  RotationSequenceAngles=[0 0 0]  RotationSequenceAnglesUnits=deg  RotationMatrix=[1 0 0; 0 1 0; 0 0 1]  BlockFunction=simmechanics.library.frames_transforms.rigid_transform
  Conn1 : PMIOPort  Port=1  Side=Right
  connections:
  Rigid Transform6/LConn1 -- Rigid Transform2/RConn1
  Rigid Transform2/LConn1 -- Rigid Transform1/LConn1 -- Rigid Transform3/RConn1
  Rigid Transform5/LConn1 -- Rigid Transform1/RConn1 -- Aesthetics/LConn1
  Conn1/RConn1 -- Rigid Transform3/LConn1
  Rail/RConn1 -- Rigid Transform6/RConn1
  Rail1/RConn1 -- Rigid Transform5/RConn1

== system SimscapeCrane_MPChard/Crane1/XY actuator/Y cart/CART ==
  BottomPlate : sm_lib/Body Elements/Solid  InertiaType=PointMass  Mass=cartMass  MassUnits=kg  CenterOfMass=[0 0 0]  CenterOfMassUnits=m  MomentsOfInertia=[1 1 1]  MomentsOfInertiaUnits=kg*m^2  ProductsOfInertia=[0 0 0]  ProductsOfInertiaUnits=kg*m^2  DensityBased=off  Density=1000  DensityUnits=kg/(m^3)  DoExposeReferenceFrame=on  SerializedFrames=<Frames/>  GraphicType=FromGeometry  MarkerShape=Sphere  MarkerSize=10  MarkerSizeUnits=m  GraphicVisPropType=SimpleVisualProperties  GraphicDiffuseColor=[1.0 1.0 1.0]  GraphicSpecularColor=[0.5 0.5 0.5 1.0]  GraphicAmbientColor=[0.15 0.15 0.15 1.0]  GraphicEmissiveColor=[0.0 0.0 0.0 1.0]  GraphicShininess=75  GraphicOpacity=0.5  GeometryShape=Brick  RectangleSize=[1 1]  RectangleSizeUnits=m  BrickDimensions=[0.18 0.2 0.02]  BrickDimensionUnits=m  CylinderRadius=1  CylinderRadiusUnits=m  CylinderLength=1  CylinderLengthUnits=m  SphereRadius=1  SphereRadiusUnits=m  EllipsoidRadii=[1 1 1]  EllipsoidRadiiUnits=m  ExtrusionCrossSection=[1 1; -1 1; -1 -1; 1 -1]  ExtrusionCrossSectionUnits=m  ExtrusionLength=1  ExtrusionLengthUnits=m  PolygonNumSides=3  PolygonOuterRadius=1  PolygonOuterRadiusUnits=m  ExtGeomFileType=STL  ExtGeomFileUnits=m  RevolutionCrossSection=[1 1; 1 -1; 2 -1; 2 1]  RevolutionCrossSectionUnits=m  RevolutionExtent=Full  RevolutionAngle=180  RevolutionAngleUnits=deg  BlockFunction=simmechanics.library.body_elements.solid
  Motor : Subsystem
  Rigid Transform1 : sm_lib/Frames and Transforms/Rigid Transform  TranslationMethod=StandardAxis  TranslationLengthUnit=m  TranslationStandardAxis=-X  TranslationStandardOffset=0.04  TranslationCartesianOffset="[-0.5 0  0]"  TranslationROffset=0  TranslationROffsetUnits=m  TranslationZOffset=0  TranslationZOffsetUnits=m  TranslationThetaOffset=0  TranslationThetaOffsetUnits=deg  RotationMethod=None  RotationAngleUnits=deg  RotationStandardAxis=-Y  RotationAngle=90  RotationArbitraryAxis=[0 0 1]  FollAlignAxisA=+X  BaseAlignAxisA=+Y  FollAlignAxisB=+Y  BaseAlignAxisB=+Z  RotationSequenceAxes=FollowerAxes  RotationSequence=XYX  RotationSequenceAngles=[0 0 0]  RotationSequenceAnglesUnits=deg  RotationMatrix=[1 0 0; 0 1 0; 0 0 1]  BlockFunction=simmechanics.library.frames_transforms.rigid_transform
  Rigid Transform2 : sm_lib/Frames and Transforms/Rigid Transform  TranslationMethod=StandardAxis  TranslationLengthUnit=m  TranslationStandardAxis=-Z  TranslationStandardOffset=0.07  TranslationCartesianOffset="[-0.5 0  0]"  TranslationROffset=0  TranslationROffsetUnits=m  TranslationZOffset=0  TranslationZOffsetUnits=m  TranslationThetaOffset=0  TranslationThetaOffsetUnits=deg  RotationMethod=None  RotationAngleUnits=deg  RotationStandardAxis=-Y  RotationAngle=90  RotationArbitraryAxis=[0 0 1]  FollAlignAxisA=+X  BaseAlignAxisA=+Y  FollAlignAxisB=+Y  BaseAlignAxisB=+Z  RotationSequenceAxes=FollowerAxes  RotationSequence=XYX  RotationSequenceAngles=[0 0 0]  RotationSequenceAnglesUnits=deg  RotationMatrix=[1 0 0; 0 1 0; 0 0 1]  BlockFunction=simmechanics.library.frames_transforms.rigid_transform
  Rigid Transform7 : sm_lib/Frames and Transforms/Rigid Transform  TranslationMethod=StandardAxis  TranslationLengthUnit=m  TranslationStandardAxis=+Z  TranslationStandardOffset=0.04  TranslationCartesianOffset="[-0.5 0  0]"  TranslationROffset=0  TranslationROffsetUnits=m  TranslationZOffset=0  TranslationZOffsetUnits=m  TranslationThetaOffset=0  TranslationThetaOffsetUnits=deg  RotationMethod=None  RotationAngleUnits=deg  RotationStandardAxis=-X  RotationAngle=90  RotationArbitraryAxis=[0 0 1]  FollAlignAxisA=+X  BaseAlignAxisA=+Y  FollAlignAxisB=+Y  BaseAlignAxisB=+Z  RotationSequenceAxes=FollowerAxes  RotationSequence=XYX  RotationSequenceAngles=[0 0 0]  RotationSequenceAnglesUnits=deg  RotationMatrix=[1 0 0; 0 1 0; 0 0 1]  BlockFunction=simmechanics.library.frames_transforms.rigid_transform
  Rigid Transform8 : sm_lib/Frames and Transforms/Rigid Transform  TranslationMethod=StandardAxis  TranslationLengthUnit=m  TranslationStandardAxis=-Y  TranslationStandardOffset=0.1  TranslationCartesianOffset="[-0.5 0  0]"  TranslationROffset=0  TranslationROffsetUnits=m  TranslationZOffset=0  TranslationZOffsetUnits=m  TranslationThetaOffset=0  TranslationThetaOffsetUnits=deg  RotationMethod=None  RotationAngleUnits=deg  RotationStandardAxis=-X  RotationAngle=90  RotationArbitraryAxis=[0 0 1]  FollAlignAxisA=+X  BaseAlignAxisA=+Y  FollAlignAxisB=+Y  BaseAlignAxisB=+Z  RotationSequenceAxes=FollowerAxes  RotationSequence=XYX  RotationSequenceAngles=[0 0 0]  RotationSequenceAnglesUnits=deg  RotationMatrix=[1 0 0; 0 1 0; 0 0 1]  BlockFunction=simmechanics.library.frames_transforms.rigid_transform
  Tower : sm_lib/Body Elements/Solid  InertiaType=PointMass  Mass=0  MassUnits=kg  CenterOfMass=[0 0 0]  CenterOfMassUnits=m  MomentsOfInertia=[1 1 1]  MomentsOfInertiaUnits=kg*m^2  ProductsOfInertia=[0 0 0]  ProductsOfInertiaUnits=kg*m^2  DensityBased=off  Density=1000  DensityUnits=kg/(m^3)  DoExposeReferenceFrame=on  SerializedFrames=<Frames/>  GraphicType=FromGeometry  MarkerShape=Sphere  MarkerSize=10  MarkerSizeUnits=m  GraphicVisPropType=SimpleVisualProperties  GraphicDiffuseColor=[1.0 1.0 1.0]  GraphicSpecularColor=[0.5 0.5 0.5 1.0]  GraphicAmbientColor=[0.15 0.15 0.15 1.0]  GraphicEmissiveColor=[0.0 0.0 0.0 1.0]  GraphicShininess=75  GraphicOpacity=0.5  GeometryShape=Brick  RectangleSize=[1 1]  RectangleSizeUnits=m  BrickDimensions=[0.06 0.12 0.12]  BrickDimensionUnits=m  CylinderRadius=1  CylinderRadiusUnits=m  CylinderLength=1  CylinderLengthUnits=m  SphereRadius=1  SphereRadiusUnits=m  EllipsoidRadii=[1 1 1]  EllipsoidRadiiUnits=m  ExtrusionCrossSection=[1 1; -1 1; -1 -1; 1 -1]  ExtrusionCrossSectionUnits=m  ExtrusionLength=1  ExtrusionLengthUnits=m  PolygonNumSides=3  PolygonOuterRadius=1  PolygonOuterRadiusUnits=m  ExtGeomFileType=STL  ExtGeomFileUnits=m  RevolutionCrossSection=[1 1; 1 -1; 2 -1; 2 1]  RevolutionCrossSectionUnits=m  RevolutionExtent=Full  RevolutionAngle=180  RevolutionAngleUnits=deg  BlockFunction=simmechanics.library.body_elements.solid
  Conn1 : PMIOPort  Port=1  Side=Right
  connections:
  Conn1/RConn1 -- Tower/RConn1 -- Rigid Transform7/LConn1 -- Rigid Transform1/LConn1
  Rigid Transform2/RConn1 -- BottomPlate/RConn1
  Rigid Transform1/RConn1 -- Rigid Transform2/LConn1
  Rigid Transform8/LConn1 -- Rigid Transform7/RConn1
  Rigid Transform8/RConn1 -- Motor/LConn1

== system SimscapeCrane_MPChard/Crane1/XY actuator/DC Y/PWM & H-Bridge1/PWM Scope ==
  Electrical Reference1 : fl_lib/Electrical/Electrical Elements/Electrical Reference
  PS-Simulink Converter 2 : nesl_utility/PS-Simulink Converter  PhysicalDomain=network_engine_domain  SubClassName=ps_output  LeftPortType=input  RightPortType=output  PseudoPeriodic=off  Frequencies=[]  Unit=V  AffineConversion=off
  PWM : Scope
  Voltage Sensor : fl_lib/Electrical/Electrical Sensors/Voltage Sensor
  u : PMIOPort  Port=1  Side=Left
  wires:
  PS-Simulink Converter 2/1 -> PWM/1
  connections:
  Voltage Sensor/RConn2 -- Electrical Reference1/LConn1
  Voltage Sensor/RConn1 -- PS-Simulink Converter 2/LConn1
  u/RConn1 -- Voltage Sensor/LConn1

== system SimscapeCrane_MPChard/Crane1/XY actuator/DC Y/PWM & H-Bridge1/REV Scope ==
  Electrical Reference1 : fl_lib/Electrical/Electrical Elements/Electrical Reference
  PS-Simulink Converter 2 : nesl_utility/PS-Simulink Converter  PhysicalDomain=network_engine_domain  SubClassName=ps_output  LeftPortType=input  RightPortType=output  PseudoPeriodic=off  Frequencies=[]  Unit=V  AffineConversion=off
  REV : Scope
  Voltage Sensor : fl_lib/Electrical/Electrical Sensors/Voltage Sensor
  u : PMIOPort  Port=1  Side=Left
  wires:
  PS-Simulink Converter 2/1 -> REV/1
  connections:
  Voltage Sensor/RConn2 -- Electrical Reference1/LConn1
  Voltage Sensor/RConn1 -- PS-Simulink Converter 2/LConn1
  u/RConn1 -- Voltage Sensor/LConn1
